simulink model "TST_StateflowLoops"  (Simulink 10.0)
settings: Solver=FixedStepDiscrete  StartTime=0.0  StopTime=10.0  FixedStep=0.02  RelTol=1e-3  EnableMultiTasking=on
settings Model: Creator=kharthforeign  LastModifiedBy=unknown
settings DataIOCC: LimitDataPoints=on  SignalLoggingSaveFormat=ModelDataLogs  SaveOutput=off  SignalLogging=off  SaveTime=off
settings OptimizationCC: BlockReduction=off  ConditionallyExecuteInputs=off  OptimizeBlockIOStorage=off  BufferReuse=off  GlobalBufferReuse=off  ExpressionFolding=off  ExpressionDepthLimit=2147483647  LocalBlockOutputs=off  InitFltsAndDblsToZero=on  OptimizeDataStoreBuffers=off  BusAssignmentInplaceUpdate=off
settings DebuggingCC: SolverPrmCheckMsg=warning  FcnCallInpInsideContextMsg=warning  StateNameClashWarn=warning
settings SFSimCC: SimParseCustomCode=off
settings GRTTargetCC: GeneratePreprocessorConditionals=Disable all
settings ConfigComp: CovExternalEMLEnable=off

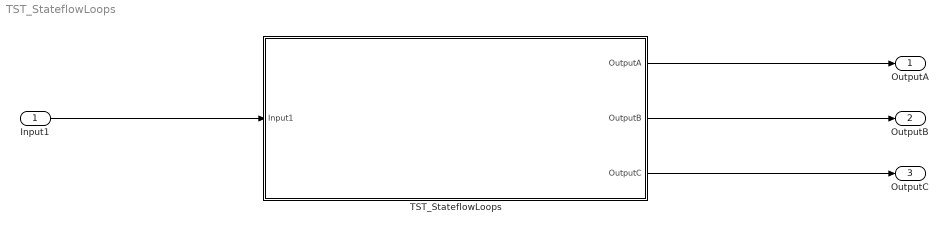
== system TST_StateflowLoops ==
  Input1 : Inport  OutDataTypeStr=uint32  BusOutputAsStruct=on
  TST_StateflowLoops : Subsystem  TreatAsAtomicUnit=on
  OutputA : Outport  OutDataTypeStr=double  PortDimensions=1
  OutputB : Outport  Port=2  OutDataTypeStr=double  PortDimensions=1
  OutputC : Outport  Port=3  OutDataTypeStr=double  PortDimensions=1
  wires:
  Input1/1 -> TST_StateflowLoops/1(Input1)
  TST_StateflowLoops/1(OutputA) -> OutputA/1
  TST_StateflowLoops/2(OutputB) -> OutputB/1
  TST_StateflowLoops/3(OutputC) -> OutputC/1

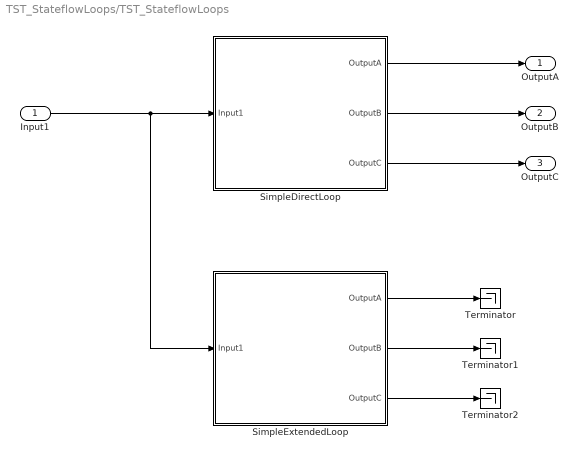
== system TST_StateflowLoops/TST_StateflowLoops ==
  Input1 : Inport  OutDataTypeStr=uint32  BusOutputAsStruct=on
  SimpleDirectLoop : Stateflow chart  TreatAsAtomicUnit=on
  SimpleExtendedLoop : Stateflow chart  TreatAsAtomicUnit=on
  Terminator : Terminator
  Terminator1 : Terminator
  Terminator2 : Terminator
  OutputA : Outport  OutDataTypeStr=double  PortDimensions=1
  OutputB : Outport  Port=2  OutDataTypeStr=double  PortDimensions=1
  OutputC : Outport  Port=3  OutDataTypeStr=double  PortDimensions=1
  wires:
  SimpleDirectLoop/1(OutputA) -> OutputA/1
  SimpleDirectLoop/2(OutputB) -> OutputB/1
  SimpleDirectLoop/3(OutputC) -> OutputC/1
  Input1/1 -> SimpleDirectLoop/1(Input1), SimpleExtendedLoop/1(Input1)
  SimpleExtendedLoop/1(OutputA) -> Terminator/1
  SimpleExtendedLoop/2(OutputB) -> Terminator1/1
  SimpleExtendedLoop/3(OutputC) -> Terminator2/1

== stateflow chart TST_StateflowLoops/SimpleDirectLoop ==
  note: simple single-transition loop
  (default) -> (junction 13) : %default
  (junction 13) -> (junction 12) [order 3] : %safe else to A
  (junction 13) -> (junction 14) [order 1] : [B]{OutputB = 1;} %else to A
  (junction 13) -> (junction 13) [order 2] : [A]{OutputA = 1;} %loop1.1
  (junction 14) -> (junction 15) [order 1] : [C]{OutputC = 1;}
  (junction 14) -> (junction 16) [order 2] : %else to C
  data: Input1 input uint32; OutputA output double =1; OutputB output double =2; OutputC output double =3; Local local uint32 =0; A local boolean; B local boolean; C local boolean

== stateflow chart TST_StateflowLoops/SimpleExtendedLoop ==
  note: loop starts at this transition
  note: simple loop consisting of several
      | transitions
  (default) -> (junction 37) : %default
  (junction 37) -> (junction 35) [order 2] : %else to A
  (junction 36) -> (junction 37) : %loop1.4
  (junction 39) -> (junction 36) [order 1] : [B]{OutputB = 1;}%loop1.3
  (junction 37) -> (junction 40) [order 1] : [A]{OutputA = 1;} %loop1.1
  (junction 39) -> (junction 38) [order 2] : %else to B
  (junction 40) -> (junction 39) : %loop1.2
  data: Input1 input uint32; OutputA output double =1; OutputB output double =2; OutputC output double =3; Local local uint32 =0; A local boolean; B local boolean; C local boolean
